simulink model "gm_DUCforLTEHDL"  (R2022b)
settings: Solver=FixedStepDiscrete  StartTime=0.0  StopTime=length(ducIn)/FsIn  RelTol=1e-3
PreLoadFcn:
  | %outputFrame = 4;
InitFcn:
  | if outputFrame == 1
  |  delay = 6;
  | else
  |  delay = 9;
  | end
undefined symbols (not defined in the file or in its folder): compFilt, FsIn, hbFilt, lowpassFilt, outputFrame, TIF
libraries: dsphdlfiltering2 x4, dspsigops x2, dsphdlsigops2 x1, dspsrcs4 x1
settings Model: Creator=The MathWorks, Inc.  LastModifiedBy=Ahmed.Soltan
settings SolverCC: AlgebraicLoopSolver=TrustRegion  MaxZcPerStep=1
settings OptimizationCC: BlockReduction=off  ConditionallyExecuteInputs=off  DefaultParameterBehavior=Inlined
settings DebuggingCC: AlgebraicLoopMsg=error  InheritedTsInSrcMsg=none  SingleTaskRateTransMsg=error  ParameterPrecisionLossMsg=none  UnconnectedInputMsg=warning  UnconnectedOutputMsg=warning  UnconnectedLineMsg=warning  SFMachineParentedDataDiag=warning
settings HardwareCC: ProdBitPerPointer=32  ProdBitPerSizeT=32  ProdBitPerPtrDiffT=32  ProdLargestAtomicFloat=None  ProdIntDivRoundTo=Undefined  ProdEndianess=Unspecified  ProdWordSize=32  ProdHWDeviceType=ASIC/FPGA->ASIC/FPGA  TargetBitPerPointer=64  TargetBitPerSizeT=64  TargetBitPerPtrDiffT=64  TargetLongLongMode=on  TargetIntDivRoundTo=Zero  TargetEndianess=LittleEndian  TargetWordSize=64  TargetHWDeviceType=Custom Processor->MATLAB Host Computer  ProdEqTarget=off
settings ModelReferenceCC: EnableRefExpFcnMdlSchedulingChecks=on
settings RTWCC: DLArmComputeVersion=19.05

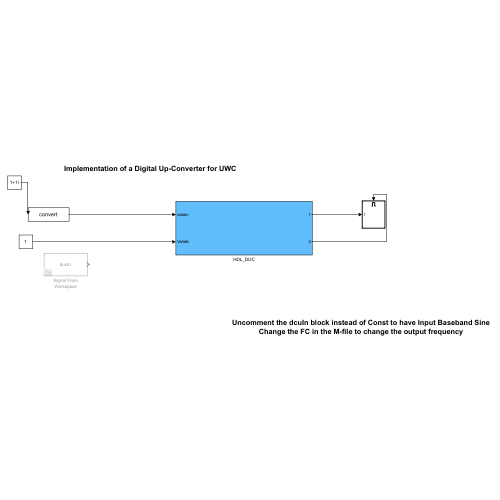
[thumbnail: Simulink's stored preview of the top-level diagram]
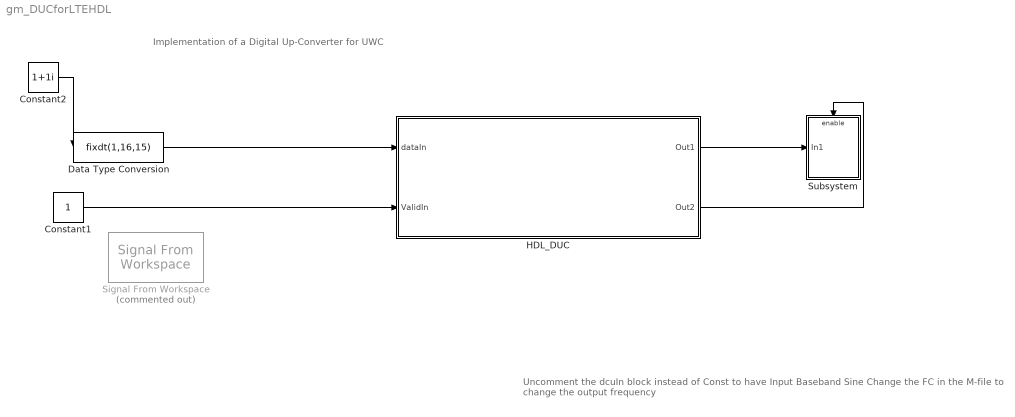
== system gm_DUCforLTEHDL ==
  note: Uncomment the dcuIn block instead of Const to have Input Baseband Sine
      | Change the FC in the M-file to change the output frequency
  note: Implementation of a Digital Up-Converter for UWC
  Constant1 : Constant  OutDataTypeStr=boolean  SampleTime=1/FsIn
  Constant2 : Constant  Value=1+1i  OutDataTypeStr=double  SampleTime=1/FsIn
  Data Type Conversion : DataTypeConversion  OutDataTypeStr=fixdt(1,16,15)  SaturateOnIntegerOverflow=off  RndMeth=Floor
  HDL_DUC : Subsystem
  Signal From Workspace : dspsrcs4/Signal From Workspace  Commented=on  X=ducIn  Ts=1/FsIn  nsamps=1  OutputAfterFinalValue=Setting to zero  ignoreOrWarnInputAndFrameLengths=off  OutputFrames=off
  Subsystem : Subsystem
  wires:
  HDL_DUC/1(Out1) -> Subsystem/1(In1)
  HDL_DUC/2(Out2) -> Subsystem/Enable
  Constant1/1 -> HDL_DUC/2(ValidIn)
  Constant2/1 -> Data Type Conversion/1
  Data Type Conversion/1 -> HDL_DUC/1(dataIn)

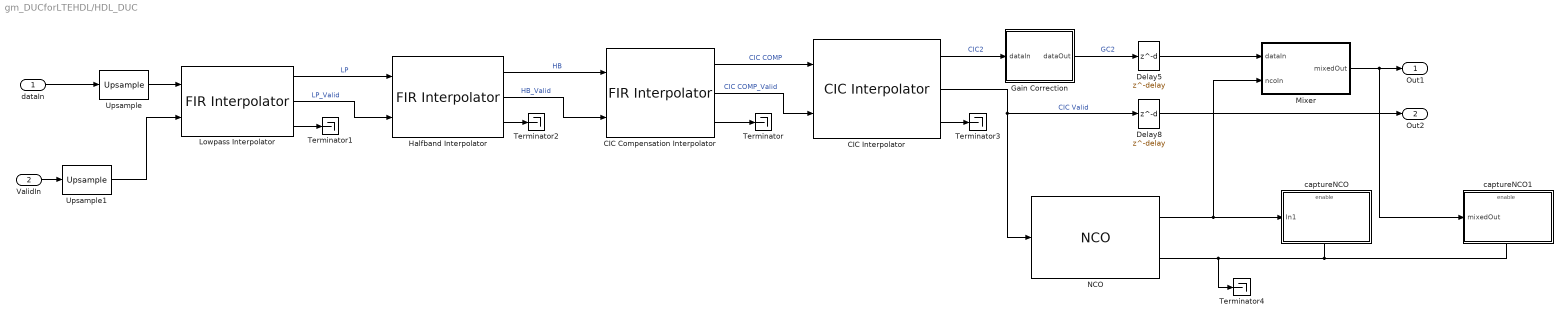
== system gm_DUCforLTEHDL/HDL_DUC ==
  dataIn : Inport
  ValidIn : Inport  Port=2
  CIC Compensation Interpolator : dsphdlfiltering2/FIR Interpolator  Numerator=compFilt.Numerator  FilterStructure=Direct form systolic  InterpolationFactor=compFilt.InterpolationFactor  NumCycles=ceil(TIF/(lowpassFilt.InterpolationFactor*hbFilt.InterpolationFactor*outputFrame))  SimulateUsing=Code generation  roundingMode=Floor  overflowMode=off  CoefficientsDataTypeStr=Inherit: Same word length as input  OutputDataTypeStr=fixdt(1,18,14)  ResetInputPort=off  HDLGlobalReset=off
  CIC Interpolator : dsphdlfiltering2/CIC Interpolator  InterpolationSource=Property  InterpolationFactor=cicFilt.InterpolationFactor  MaxInterpolationFactor=8  DifferentialDelay=1  NumSections=3  NumCycles=ceil(TIF/(lowpassFilt.InterpolationFactor*hbFilt.InterpolationFactor*compFilt.InterpolationFactor*outputFrame))  GainCorrection=off  SimulateUsing=Code generation  OutputDataType=Minimum section word lengths  OutputWordLength=18  ResetInputPort=off  HDLGlobalReset=off
  Delay5 : Delay  DelayLength=delay  InitialCondition=0
  Delay8 : Delay  DelayLength=delay  InitialCondition=0
  Gain Correction : Subsystem
  Halfband Interpolator : dsphdlfiltering2/FIR Interpolator  Numerator=hbFilt.Numerator  FilterStructure=Direct form systolic  InterpolationFactor=hbFilt.InterpolationFactor  NumCycles=ceil(TIF/(lowpassFilt.InterpolationFactor*outputFrame))  SimulateUsing=Code generation  roundingMode=Floor  overflowMode=off  CoefficientsDataTypeStr=Inherit: Same word length as input  OutputDataTypeStr=fixdt(1,18,14)  ResetInputPort=off  HDLGlobalReset=off
  Lowpass Interpolator : dsphdlfiltering2/FIR Interpolator  Numerator=lowpassFilt.Numerator  FilterStructure=Direct form systolic  InterpolationFactor=lowpassFilt.InterpolationFactor  NumCycles=ceil(TIF/outputFrame)  SimulateUsing=Code generation  roundingMode=Floor  overflowMode=off  CoefficientsDataTypeStr=Inherit: Same word length as input  OutputDataTypeStr=fixdt(1,18,14)  ResetInputPort=off  HDLGlobalReset=off
  Mixer : Subsystem
  NCO : dsphdlsigops2/NCO  PhaseIncrementSource=Property  PhaseIncrement=nco.PhaseInc  PhaseOffsetSource=Property  PhaseOffset=0  DitherSource=Property  NumDitherBits=nco.NumDitherBits  SamplesPerFrame=outputFrame  LUTCompress=on  ResetAction=off  Waveform=Complex exponential  PhasePort=off  SimulateUsing=Code generation  AccumulatorWL=nco.AccWL  PhaseQuantization=on  NumQuantizerAccumulatorBits=nco.QuantAccWL  OutputDataType=Binary point scaling  OutputWL=18  OutputFL=16
  Terminator{,1..4} (5 alike) : Terminator
  Upsample : dspsigops/Upsample  N=16  phase=0  RateOptions=Allow multirate processing  ic=0  mode=Unused parameter value
  Upsample1 : dspsigops/Upsample  N=16  phase=0  RateOptions=Allow multirate processing  ic=0  mode=Unused parameter value
  captureNCO : Subsystem
  captureNCO1 : Subsystem
  Out1 : Outport
  Out2 : Outport  Port=2
  wires:
  Upsample1/1 -> Lowpass Interpolator/2
  ValidIn/1 -> Upsample1/1
  Upsample/1 -> Lowpass Interpolator/1
  dataIn/1 -> Upsample/1
  CIC Interpolator/3 -> Terminator3/1
  Lowpass Interpolator/3 -> Terminator1/1
  Halfband Interpolator/3 -> Terminator2/1
  CIC Compensation Interpolator/3 -> Terminator/1
  Mixer/1(mixedOut) -> Out1/1, captureNCO1/1(mixedOut)
  Delay5/1 -> Mixer/1(dataIn)
  NCO/2 -> captureNCO/Enable, captureNCO1/Enable, Terminator4/1
  NCO/1 -> captureNCO/1(In1), Mixer/2(ncoIn)
  Delay8/1 -> Out2/1
  Gain Correction/1(dataOut) -> Delay5/1  "GC2"
  CIC Interpolator/1 -> Gain Correction/1(dataIn)  "CIC2"
  CIC Interpolator/2 -> Delay8/1, NCO/1  "CIC Valid"
  CIC Compensation Interpolator/2 -> CIC Interpolator/2  "CIC COMP_Valid"
  CIC Compensation Interpolator/1 -> CIC Interpolator/1  "CIC COMP"
  Halfband Interpolator/2 -> CIC Compensation Interpolator/2  "HB_Valid"
  Halfband Interpolator/1 -> CIC Compensation Interpolator/1  "HB"
  Lowpass Interpolator/2 -> Halfband Interpolator/2  "LP_Valid"
  Lowpass Interpolator/1 -> Halfband Interpolator/1  "LP"

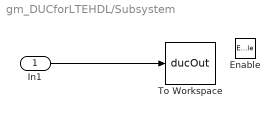
== system gm_DUCforLTEHDL/Subsystem ==
  In1 : Inport
  Enable : EnablePort
  To Workspace : ToWorkspace  VariableName=ducOut  SampleTime=-1
      settings: Save2DSignal=2-D array (concatenate along first dimension)
  wires:
  In1/1 -> To Workspace/1

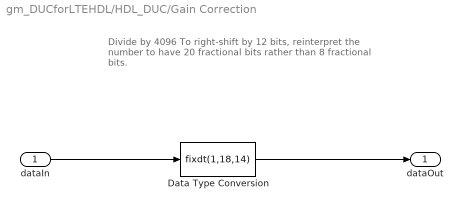
== system gm_DUCforLTEHDL/HDL_DUC/Gain Correction ==
  note: Divide by 4096
      | To right-shift by 12 bits, reinterpret the number to have
      | 20 fractional bits rather than 8 fractional bits.
  dataIn : Inport
  Data Type Conversion : DataTypeConversion  OutDataTypeStr=fixdt(1,18,14)  ConvertRealWorld=Stored Integer (SI)  SaturateOnIntegerOverflow=off  RndMeth=Floor
  dataOut : Outport  VectorParamsAs1DForOutWhenUnconnected=off
  wires:
  Data Type Conversion/1 -> dataOut/1
  dataIn/1 -> Data Type Conversion/1

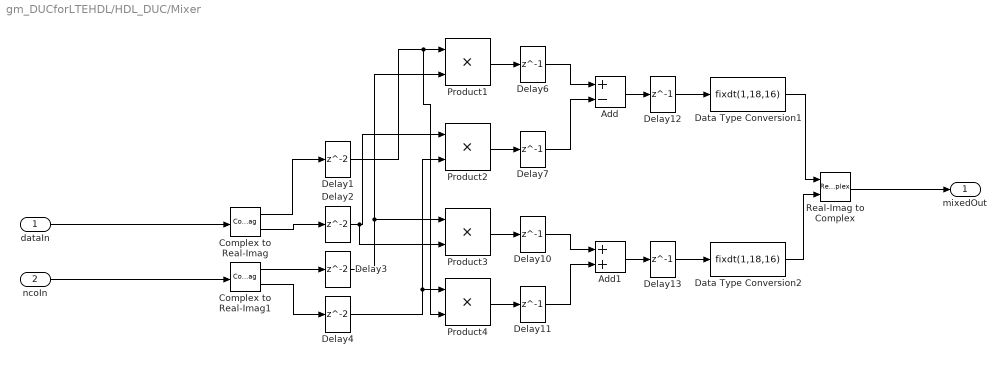
== system gm_DUCforLTEHDL/HDL_DUC/Mixer ==
  dataIn : Inport
  ncoIn : Inport  Port=2
  Add : Sum  Inputs=+-
  Add1 : Sum
  Complex to Real-Imag : ComplexToRealImag
  Complex to Real-Imag1 : ComplexToRealImag
  Data Type Conversion1 : DataTypeConversion  OutDataTypeStr=fixdt(1,18,16)  SaturateOnIntegerOverflow=off  RndMeth=Floor
  Data Type Conversion2 : DataTypeConversion  OutDataTypeStr=fixdt(1,18,16)  SaturateOnIntegerOverflow=off  RndMeth=Floor
  Delay{1..4} (4 alike) : Delay  InitialCondition=0
  Delay{6..7,10..13} (6 alike) : Delay  DelayLength=1  InitialCondition=0
  Product{1..4} (4 alike) : Product
  Real-Imag to Complex : RealImagToComplex
  mixedOut : Outport
  wires:
  Product4/1 -> Delay11/1
  Product3/1 -> Delay10/1
  Data Type Conversion1/1 -> Real-Imag to Complex/1
  Complex to Real-Imag/2 -> Delay2/1
  Delay3/1 -> Product3/1, Product1/2
  Add1/1 -> Delay13/1
  Complex to Real-Imag1/1 -> Delay3/1
  dataIn/1 -> Complex to Real-Imag/1
  Real-Imag to Complex/1 -> mixedOut/1
  Delay2/1 -> Product3/2, Product2/1
  Delay12/1 -> Data Type Conversion1/1
  Delay4/1 -> Product4/1, Product2/2
  Add/1 -> Delay12/1
  Delay13/1 -> Data Type Conversion2/1
  Delay6/1 -> Add/1
  Data Type Conversion2/1 -> Real-Imag to Complex/2
  Complex to Real-Imag/1 -> Delay1/1
  Complex to Real-Imag1/2 -> Delay4/1
  Delay7/1 -> Add/2
  Product2/1 -> Delay7/1
  Product1/1 -> Delay6/1
  ncoIn/1 -> Complex to Real-Imag1/1
  Delay1/1 -> Product4/2, Product1/1
  Delay11/1 -> Add1/2
  Delay10/1 -> Add1/1

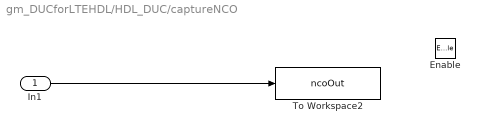
== system gm_DUCforLTEHDL/HDL_DUC/captureNCO ==
  In1 : Inport
  Enable : EnablePort
  To Workspace2 : ToWorkspace  VariableName=ncoOut  SampleTime=-1
      settings: Save2DSignal=2-D array (concatenate along first dimension)
  wires:
  In1/1 -> To Workspace2/1

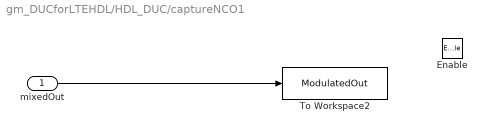
== system gm_DUCforLTEHDL/HDL_DUC/captureNCO1 ==
  mixedOut : Inport
  Enable : EnablePort
  To Workspace2 : ToWorkspace  VariableName=ModulatedOut  SampleTime=-1
      settings: Save2DSignal=2-D array (concatenate along first dimension)
  wires:
  mixedOut/1 -> To Workspace2/1
